simulink model "Lab10"  (R2022a)
settings: Solver=ode23  StartTime=0.0  StopTime=50  FixedStep=1e-4  MaxStep=1e-4  RelTol=1e-4
model workspace (MAT data in the model file):
  L = 2
  Sig = Simulink.Signal
  Sig.DataType = 'auto'
  Sig.Dimensions = -1
  Sig.DimensionsMode = 'auto'
  Sig.Complexity = 'auto'
  Sig.SampleTime = -1
  Sig.SamplingMode = 'auto'
  g = 9.8
  mC = 10
  mL = 20
undefined symbols (not defined in the file): sigbuilder_block
libraries: dspsrcs4 x3, simulink x1
settings Model: PacingRate=1.100000  Creator=ishaan  LastModifiedBy=ishaan
settings SolverCC: ZeroCrossAlgorithm=Adaptive
settings DataIOCC: ExternalInput=tspan  SaveState=on  LoggingToFile=on

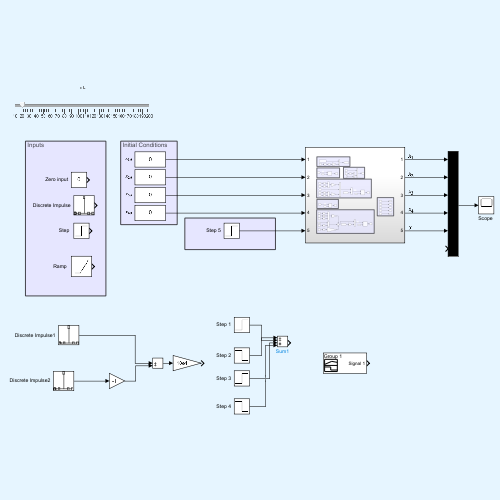
[thumbnail: Simulink's stored preview of the top-level diagram]
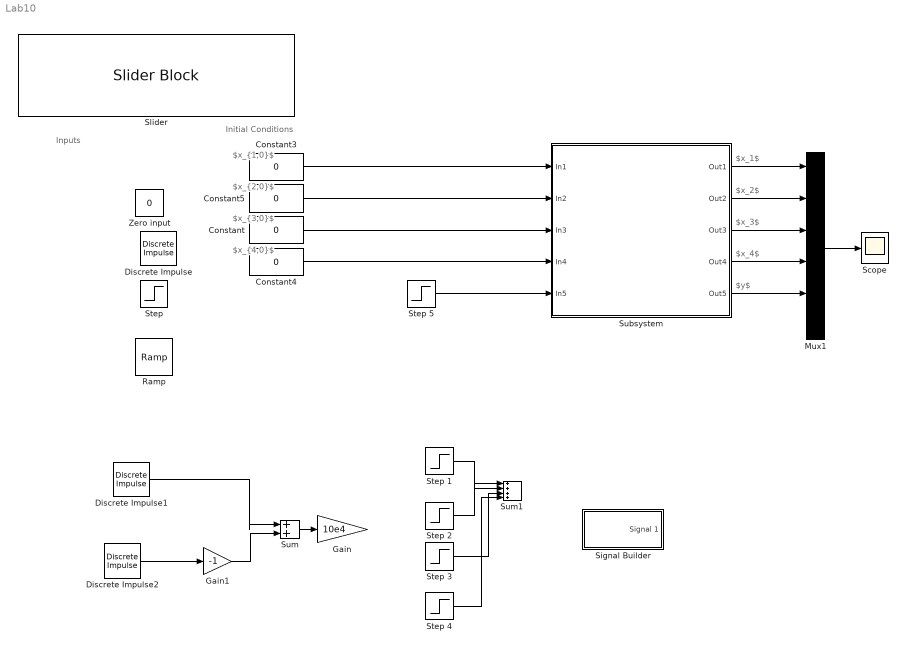
== system Lab10 ==
  note: $x_1$
  note: $x_{1,0}$
  note: Initial Conditions
  note: Inputs
  note: $x_{2,0}$
  note: $x_{3,0}$
  note: $x_{4,0}$
  note: $x_2$
  note: $x_3$
  note: $x_4$
  note: $y$
  Constant{,3..5} (4 alike) : Constant  Value=0
  Discrete Impulse : dspsrcs4/Discrete  Impulse  Delay=0  SampleTime=1e-4  FrameSample=1  OutputFrames=off  dataType=double  isSigned=on  wordLen=16  udDataType=sfix(16)  fracBitsMode=Best precision  numFracBits=15  OutDataTypeStr=double  LastOutDataTypeStr=double
  Discrete Impulse1 : dspsrcs4/Discrete  Impulse  Delay=0  SampleTime=1e-4  FrameSample=1  OutputFrames=off  dataType=double  isSigned=on  wordLen=16  udDataType=sfix(16)  fracBitsMode=Best precision  numFracBits=15  OutDataTypeStr=double  LastOutDataTypeStr=double
  Discrete Impulse2 : dspsrcs4/Discrete  Impulse  Delay=50000  SampleTime=1e-4  FrameSample=1  OutputFrames=off  dataType=double  isSigned=on  wordLen=16  udDataType=sfix(16)  fracBitsMode=Best precision  numFracBits=15  OutDataTypeStr=double  LastOutDataTypeStr=double
  Gain : Gain  Gain=10e4
  Gain1 : Gain  Gain=-1
  Mux1 : Mux  Inputs=6
  "Ramp " : simulink/Sources/Ramp  slope=1  start=0  InitialOutput=0
  "Scope " : Scope
  Signal Builder : Subsystem  Tag=STV Subsys  LoadFcn=sigbuilder_block('load');  StartFcn=sigbuilder_block('start');  StopFcn=sigbuilder_block('stop');  ClipboardFcn=sigbuilder_block('clipboard');  mask(Sigbuilder block){tuvar=[0:10]}
      mask help: Simulink:masks:SigbuilderBlock_MD
      mask init:
      | if ~strcmp(get_param(bdroot(gcbh),'SimulationStatus'),'stopped') tuvar = sigbuilder_block('maskInit'); end
      settings: CopyFcn=sigbuilder_block('copy');  DeleteFcn=sigbuilder_block('delete');  ModelCloseFcn=sigbuilder_block('modelClose');  PreSaveFcn=sigbuilder_block('preSave');  PauseFcn=sigbuilder_block('pause');  ContinueFcn=sigbuilder_block('continue');  NameChangeFcn=sigbuilder_block('namechange');  OpenFcn=sigbuilder_block('open',[0 30 1152 561.6 ]);  CloseFcn=sigbuilder_block('close');
      mask Display: plot(0, 0, 100, 100,[2, 2, 32, 32, 2], [68, 8, 8, 68, 68],[32, 2], [38, 38], [32, 19, 2],[53, 60, 44], [32, 17, 17, 2],[16, 16, 31, 31]);txt = getActiveGroup(gcbh);text(2, 100, txt,'verticalAlignment', 'top');
  Slider : SliderBlock  ScaleMin=10  ScaleMax=200
  "Step " : Step  Time=0  SampleTime=0
  Step 1 : Step  Time=0  SampleTime=0
  Step 2 : Step  Time=10  After=-1  SampleTime=0
  Step 3 : Step  Time=15  After=+1  SampleTime=0
  Step 4 : Step  Time=5  After=-1  SampleTime=0
  Step 5 : Step  Time=0  SampleTime=0
  Subsystem : Subsystem
  Sum : Sum  Inputs=|++
  Sum1 : Sum  Inputs=++++
  Zero input : Constant  Value=0
  wires:
  Mux1/1 -> "Scope "/1
  Constant3/1 -> Subsystem/1(In1)
  Constant5/1 -> Subsystem/2(In2)
  Constant/1 -> Subsystem/3(In3)
  Constant4/1 -> Subsystem/4(In4)
  Subsystem/1(Out1) -> Mux1/1
  Subsystem/2(Out2) -> Mux1/2
  Subsystem/3(Out3) -> Mux1/3
  Subsystem/4(Out4) -> Mux1/4
  Subsystem/5(Out5) -> Mux1/5
  Discrete Impulse2/1 -> Gain1/1
  Discrete Impulse1/1 -> Sum/1
  Gain1/1 -> Sum/2
  Sum/1 -> Gain/1
  Step 1/1 -> Sum1/2
  Step 2/1 -> Sum1/1
  Step 3/1 -> Sum1/3
  Step 4/1 -> Sum1/4
  Step 5/1 -> Subsystem/5(In5)

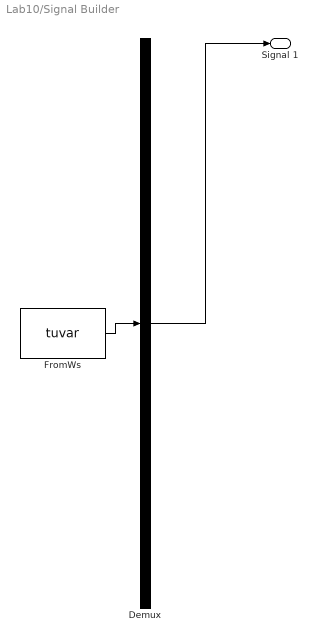
== system Lab10/Signal Builder ==
  Demux : Demux  Tag=STV Demux  Outputs=1
      settings: DisplayOption=none
  FromWs : FromWorkspace  Tag=STV FromWs  VariableName=tuvar
      SigBuilderData=|
      | common.afterFinalStr = 'Extrapolate'
      | common.sampleTime = '0'
      | dataSet.timeRange = [0 50]
      | dataSet.name = 'Group 1'
      | sbobj.Groups.Name = 'Group 1'
      | sbobj.Groups.Signals.Name = 'Signal 1'
      | sbobj.Groups.Signals.XData = [0 10 15 25 50]
      | sbobj.Groups.Signals.YData = [0 1.01 -1 0 0]
      | sbobj.Groups.TimeRange = [0 50]
  Signal 1 : Outport  Tag=STV Outport
  wires:
  Demux/1 -> Signal 1/1
  FromWs/1 -> Demux/1

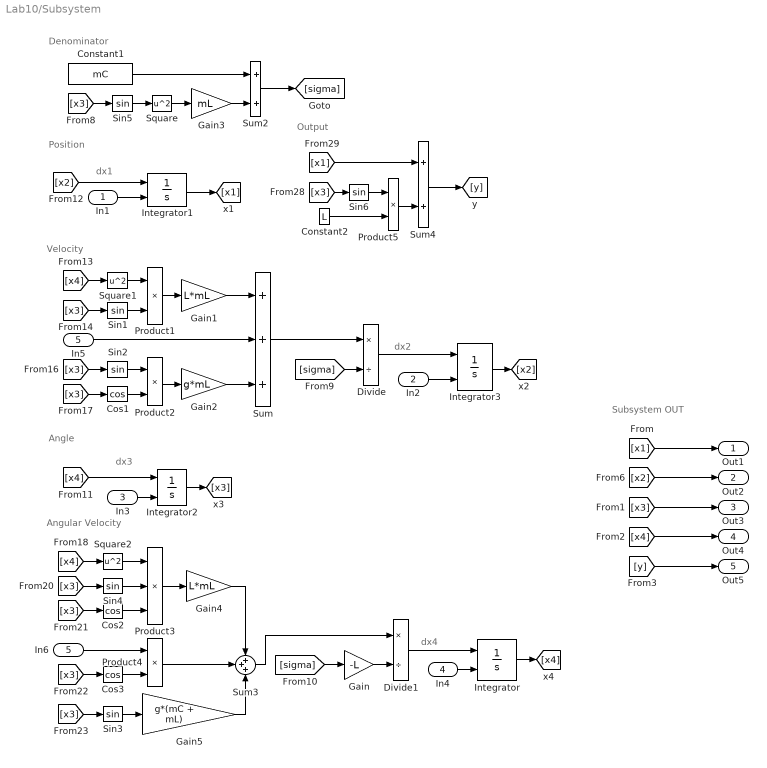
== system Lab10/Subsystem ==
  note: Subsystem OUT
  note: dx4
  note: dx2
  note: dx1
  note: dx3
  note: Denominator
  note: Output
  note: Position
  note: Angle
  note: Velocity
  note: Angular Velocity
  In1 : Inport
  In2 : Inport  Port=2
  In3 : Inport  Port=3
  In4 : Inport  Port=4
  In5 : Inport  Port=5
  Constant1 : Constant  Value=mC
  Constant2 : Constant  Value=L
  Cos1 : Trigonometry  Operator=cos
  Cos2 : Trigonometry  Operator=cos
  Cos3 : Trigonometry  Operator=cos
  Divide : Product  Inputs=*/
  Divide1 : Product  Inputs=*/
  Gain : Gain  Gain=-L
  Gain1 : Gain  Gain=L*mL
  Gain2 : Gain  Gain=g*mL
  Gain3 : Gain  Gain=mL
  Gain4 : Gain  Gain=L*mL
  Gain5 : Gain  Gain=g*(mC + mL)
  In6 : InportShadow  Port=5
  Integrator : Integrator  InitialConditionSource=external
  Integrator1 : Integrator  InitialConditionSource=external
  Integrator2 : Integrator  InitialConditionSource=external  InitialCondition=pi+0.01  WrappedStateUpperValue=2*pi  WrappedStateLowerValue=0
  Integrator3 : Integrator  InitialConditionSource=external
  Product{1..2,4..5} (4 alike) : Product
  Product3 : Product  Inputs=3
  Sin{1..6} (6 alike) : Trigonometry
  Square : Math  Operator=square
  Square1 : Math  Operator=square
  Square2 : Math  Operator=square
  Sum : Sum  Inputs=+++
  Sum2 : Sum
  Sum3 : Sum  Inputs=+++
  Sum4 : Sum
  Out1 : Outport
  Out2 : Outport  Port=2
  Out3 : Outport  Port=3
  Out4 : Outport  Port=4
  Out5 : Outport  Port=5
  wires:
  Sum4/1 -> [y]
  [y] -> Out5/1
  [x2] -> Integrator1/1
  [x3] -> Sin2/1
  Sin1/1 -> Product1/2
  Sum2/1 -> [sigma]
  Sum3/1 -> Divide1/1
  Product2/1 -> Gain2/1
  [x3] -> Cos3/1
  [x2] -> Out2/1
  Gain3/1 -> Sum2/2
  Divide1/1 -> Integrator/1
  [x3] -> Sin4/1
  In1/1 -> Integrator1/2
  Gain5/1 -> Sum3/3
  [sigma] -> Divide/2
  Product5/1 -> Sum4/2
  Constant2/1 -> Product5/2
  Square/1 -> Gain3/1
  Sin6/1 -> Product5/1
  Sin3/1 -> Gain5/1
  Integrator2/1 -> [x3]
  Cos1/1 -> Product2/2
  Gain4/1 -> Sum3/1
  [sigma] -> Gain/1
  [x4] -> Out4/1
  Square1/1 -> Product1/1
  [x3] -> Sin1/1
  Sum/1 -> Divide/1
  Product1/1 -> Gain1/1
  [x3] -> Cos2/1
  [x4] -> Square1/1
  Product3/1 -> Gain4/1
  [x3] -> Cos1/1
  [x1] -> Sum4/1
  In2/1 -> Integrator3/2
  [x3] -> Out3/1
  Sin4/1 -> Product3/2
  Sin2/1 -> Product2/1
  Gain2/1 -> Sum/3
  Gain/1 -> Divide1/2
  [x1] -> Out1/1
  Integrator/1 -> [x4]
  [x3] -> Sin6/1
  Constant1/1 -> Sum2/1
  Cos3/1 -> Product4/2
  Gain1/1 -> Sum/1
  [x4] -> Integrator2/1
  [x3] -> Sin5/1
  [x4] -> Square2/1
  In3/1 -> Integrator2/2
  In4/1 -> Integrator/2
  Cos2/1 -> Product3/3
  Square2/1 -> Product3/1
  [x3] -> Sin3/1
  Divide/1 -> Integrator3/1
  Integrator3/1 -> [x2]
  Product4/1 -> Sum3/2
  Integrator1/1 -> [x1]
  Sin5/1 -> Square/1
  In5/1 -> Sum/2
  In6/1 -> Product4/1
